simulink model "ECO_openSource"  (R2020b)
settings: Solver=FixedStepAuto  StartTime=0.0  StopTime=parECO.ref.time(end)+parECO.ref.dT  FixedStep=0.001  RelTol=1e-3  EnableMultiTasking=on
InitFcn:
  | if ~exist('parECO','var')
  |    load('parECO.mat');
  | end
  | if ~isfield(parECO,'ref')
  | 
  |    parECO.enNoise = true;
  |    parECO.enDist = true;
  |    parECO.enFB.imep = true;
  |    parECO.enFB.dpMax = true;
  |    parECO.enFB.Tevo = true;
  |    parECO.enFB.cNOx = true;
  | 
  |    parECO.ref.dT = 5;
  |    parECO.ref.imep = [  6   6   9   9   7   7 ] * 1e5
  |    parECO.ref.dpMax = [ 15   4   4   4   4   4 ] * 1e5;
  |    parECO.ref.Tevo = [  0   0   0 680   0   0 ] + 273;
  |    parECO.ref.cNOx = [100 100 100 100 100  15 ] * 1e2;
  | 
  |    parECO.ref.time  = 0 : parECO.ref.dT : parECO.ref.dT*(numel(parECO.ref.imep)-1);
  |    parECO.ref.imep  = [parECO.Reference.IMEP parECO.ref.imep(1)  parECO.ref.imep ];
  |    parECO.ref.dpMax = [parECO.Reference.dpMax parECO.ref.dpMax(1) parECO.ref.dpMax];
  |    parECO.ref.Tevo  = [parECO.Reference.Tmin parECO.ref.Tevo(1)  parECO.ref.Tevo];
  |    parECO.ref.cNOx  = [parECO.Reference.cNOx parECO.ref.cNOx(1)  parECO.ref.cNOx];
  |    parECO.ref.time  = [0 1 parECO.ref.time + parECO.ref.dT ];
  | 
  | end
undefined symbols (not defined in the file): DiscIntNeverNeededParam, parOpt, parSim
libraries: simulink x6, dspstat3 x4, dspswit3 x1, hdlsllib x1
(part 1 of 2)
settings Model: NumberOfSteps=5000  Creator=shaen  LastModifiedBy=nicolas
settings DataIOCC: ReturnWorkspaceOutputs=off
settings DebuggingCC: InheritedTsInSrcMsg=none  ArithmeticOperatorsInVariantConditions=warning
settings SFSimCC: SimUseLocalCustomCode=off  CustomCodeUndefinedFunction=UseInterfaceOnly
settings RTWCC: RTWUseLocalCustomCode=off

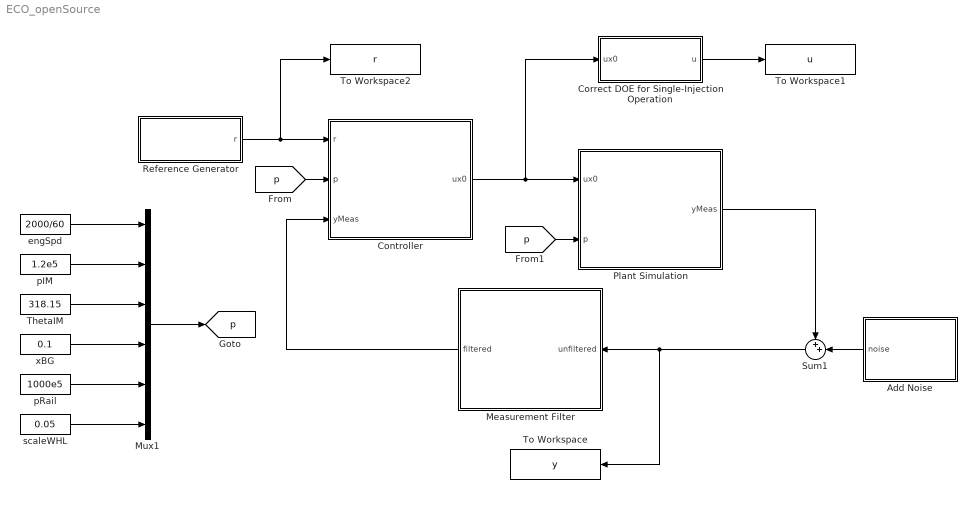
== system ECO_openSource ==
  Add Noise : Subsystem
  Controller : Subsystem  Description=test
  Correct DOE for Single-Injection Operation : Subsystem
  Measurement Filter : Subsystem
  Mux1 : Mux  Inputs=6
  Plant Simulation : Subsystem
  Reference Generator : Subsystem
  Sum1 : Sum  Inputs=++|
  ThetaIM : Constant  Value=318.15
  To Workspace : ToWorkspace  VariableName=y  SaveFormat=Timeseries  SampleTime=-1
  To Workspace1 : ToWorkspace  VariableName=u  SaveFormat=Timeseries  SampleTime=-1
  To Workspace2 : ToWorkspace  VariableName=r  SaveFormat=Timeseries  SampleTime=-1
  engSpd : Constant  Value=2000/60
  pIM : Constant  Value=1.2e5
  pRail : Constant  Value=1000e5
  scaleWHL : Constant  Value=0.05
  xBG : Constant  Value=0.1
  tag scope: p=global
  wires:
  [p] -> Plant Simulation/2(p)
  Reference Generator/1(r) -> To Workspace2/1, Controller/1(r)
  Sum1/1 -> To Workspace/1, Measurement Filter/1(unfiltered)
  pRail/1 -> Mux1/5
  Plant Simulation/1(yMeas) -> Sum1/1
  Mux1/1 -> [p]
  Correct DOE for Single-Injection Operation/1(" u ") -> To Workspace1/1
  ThetaIM/1 -> Mux1/3
  Measurement Filter/1(filtered) -> Controller/3(yMeas)
  scaleWHL/1 -> Mux1/6
  Add Noise/1(noise) -> Sum1/2
  pIM/1 -> Mux1/2
  xBG/1 -> Mux1/4
  [p] -> Controller/2(p)
  engSpd/1 -> Mux1/1
  Controller/1(ux0) -> Correct DOE for Single-Injection Operation/1(ux0), Plant Simulation/1(ux0)

== system ECO_openSource/Add Noise ==
  Gain1 : Gain  Gain=0.25*1e4
  Gain2 : Gain  Gain=2
  Gain3 : Gain  Gain=2
  Gain4 : Gain  Gain=0.15*1e5
  Mux7 : Mux
  ON/OFF : Gain  Gain=parECO.enNoise
  Random Number1 : RandomNumber  SampleTime=0.01
  Random Number2 : RandomNumber  Seed=1  SampleTime=0.01
  Random Number3 : RandomNumber  Seed=2  SampleTime=0.01
  Random Number4 : RandomNumber  Seed=1  SampleTime=0.01
  noise : Outport
  wires:
  Random Number3/1 -> Gain4/1
  Mux7/1 -> ON/OFF/1
  Random Number2/1 -> Gain3/1
  ON/OFF/1 -> noise/1
  Random Number1/1 -> Gain1/1
  Gain1/1 -> Mux7/1
  Gain4/1 -> Mux7/4
  Gain3/1 -> Mux7/3
  Random Number4/1 -> Gain2/1
  Gain2/1 -> Mux7/2

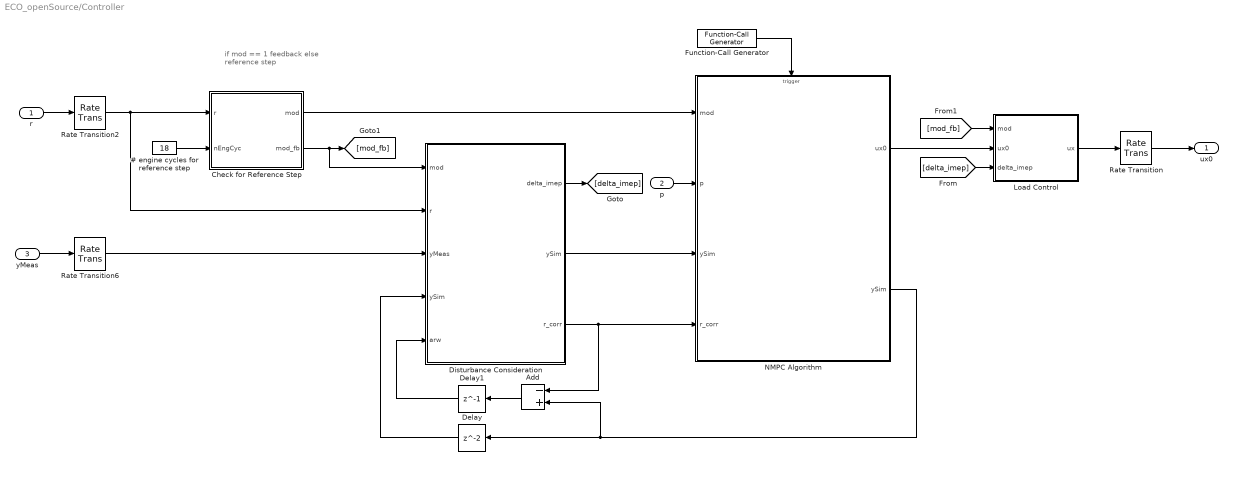
== system ECO_openSource/Controller ==
  note: if mod == 1
      | 	feedback
      | else
      | 	reference step
  r : Inport
  p : Inport  Port=2
  yMeas : Inport  Port=3
  # engine cycles for reference step : Constant  Value=18
  Add : Sum  Inputs=-+
  Check for Reference Step : Subsystem
  Delay : Delay  InitialCondition=repmat([parECO.Reference.IMEP;parECO.Reference.cNOx;parECO.Reference.Tmin;parECO.Reference.dpMax],1,2)
  Delay1 : Delay  DelayLength=1
  Disturbance Consideration : Subsystem
  Function-Call Generator : simulink/Ports & Subsystems/Function-Call Generator  sample_time=parECO.T_ECO  numberOfIterations=1  DisallowWideOutput=off
  Load Control : Subsystem
  NMPC Algorithm : Subsystem
  Rate Transition : RateTransition  InitialCondition=parECO.ux0
  Rate Transition2 : RateTransition  InitialCondition=[parECO.Reference.IMEP;parECO.Reference.cNOx;parECO.Reference.Tmin;parECO.Reference.dpMax]
  Rate Transition6 : RateTransition
  ux0 : Outport  VectorParamsAs1DForOutWhenUnconnected=off
  wires:
  Rate Transition/1 -> ux0/1
  Function-Call Generator/1 -> NMPC Algorithm/Trigger
  yMeas/1 -> Rate Transition6/1
  # engine cycles for reference step/1 -> Check for Reference Step/2(nEngCyc)
  Check for Reference Step/1(mod) -> NMPC Algorithm/1(mod)
  Rate Transition6/1 -> Disturbance Consideration/3(yMeas)
  r/1 -> Rate Transition2/1
  NMPC Algorithm/1(ux0) -> Load Control/2(ux0)
  Rate Transition2/1 -> Disturbance Consideration/2(r), Check for Reference Step/1(r)
  Add/1 -> Delay1/1
  Delay/1 -> Disturbance Consideration/4(ySim)
  Disturbance Consideration/2(" ySim ") -> NMPC Algorithm/3(" ySim ")
  Disturbance Consideration/3(r_corr) -> Add/1, NMPC Algorithm/4(r_corr)
  Load Control/1(ux) -> Rate Transition/1
  Disturbance Consideration/1(delta_imep) -> [delta_imep]
  [delta_imep] -> Load Control/3(delta_imep)
  Check for Reference Step/2(mod_fb) -> Disturbance Consideration/1(mod), [mod_fb]
  [mod_fb] -> Load Control/1(mod)
  Delay1/1 -> Disturbance Consideration/5(arw)
  p/1 -> NMPC Algorithm/2(p)
  NMPC Algorithm/2(ySim) -> Add/2, Delay/1

== system ECO_openSource/Correct DOE for Single-Injection Operation ==
  ux0 : Inport
  MATLAB Function : MATLAB Function  TreatAsAtomicUnit=on
  Selector : Selector  InputPortWidth=10  IndexOptions=Index vector (dialog)  Indices=1:4  OutputSizes=1
  " u " : Outport
  wires:
  ux0/1 -> Selector/1
  MATLAB Function/1(u) -> " u "/1
  Selector/1 -> MATLAB Function/1("u ")

== system ECO_openSource/Measurement Filter ==
  unfiltered : Inport
  Demux : Demux
  Moving Average{,1..3} (4 alike) : dspstat3/Moving Average  Method=Sliding window  SpecifyWindowLength=on  WindowLength=4  ForgettingFactor=0.9  SimulateUsing=Code generation
  Mux7 : Mux
  filtered : Outport
  wires:
  unfiltered/1 -> Demux/1
  Mux7/1 -> filtered/1
  Demux/1 -> Moving Average/1
  Moving Average/1 -> Mux7/1
  Demux/2 -> Moving Average1/1
  Moving Average1/1 -> Mux7/2
  Demux/3 -> Moving Average2/1
  Moving Average2/1 -> Mux7/3
  Demux/4 -> Moving Average3/1
  Moving Average3/1 -> Mux7/4

== system ECO_openSource/Plant Simulation ==
  ux0 : Inport
  p : Inport  Port=2
  Create Measurements : Subsystem
  Delay1 : Delay  DelayLength=1  InitialConditionSource=Input port  InitialCondition=[parOpt.u0;parSim.OP.pInt;0;0]
      settings: InputPortMap=u0,p4
  For Iterator : ForIterator  ResetStates=reset  IterationLimit=numel(parECO.ca_sim)-1  ShowIterationPort=off
  S-Function : S-Function  FunctionName=sfun_fsim  SFunctionDeploymentMode=off  EnableBusSupport=off
  dca : Constant  Value=parECO.dca_sim
  yMeas : Outport
  wires:
  S-Function/1 -> Delay1/1, Create Measurements/1(ux)  "ux"
  Delay1/1 -> S-Function/1
  Create Measurements/1(yMeas) -> yMeas/1
  S-Function/2 -> Create Measurements/2(uxdot)  "uxdot"
  S-Function/3 -> Create Measurements/3(y)  "y"
  ux0/1 -> Delay1/2
  dca/1 -> S-Function/3
  p/1 -> S-Function/2

== system ECO_openSource/Reference Generator ==
  1-D Lookup Table : Lookup_n-D  NumberOfTableDimensions=1  BreakpointsForDimension1=parECO.ref.time  Table=parECO.ref.imep  InterpMethod=Flat  ExtrapMethod=Clip  InternalRulePriority=Speed  RndMeth=Simplest  InputSameDT=on
  1-D Lookup Table1 : Lookup_n-D  NumberOfTableDimensions=1  BreakpointsForDimension1=parECO.ref.time  Table=parECO.ref.Tevo  InterpMethod=Flat  ExtrapMethod=Clip  InternalRulePriority=Speed  RndMeth=Simplest  InputSameDT=on
  1-D Lookup Table2 : Lookup_n-D  NumberOfTableDimensions=1  BreakpointsForDimension1=parECO.ref.time  Table=parECO.ref.dpMax  InterpMethod=Flat  ExtrapMethod=Clip  InternalRulePriority=Speed  RndMeth=Simplest  InputSameDT=on
  1-D Lookup Table3 : Lookup_n-D  NumberOfTableDimensions=1  BreakpointsForDimension1=parECO.ref.time  Table=parECO.ref.cNOx  InterpMethod=Flat  ExtrapMethod=Clip  InternalRulePriority=Speed  RndMeth=Simplest  InputSameDT=on
  Clock : Clock
  Mux : Mux
  r : Outport  VectorParamsAs1DForOutWhenUnconnected=off
  wires:
  1-D Lookup Table/1 -> Mux/1
  Mux/1 -> r/1
  Clock/1 -> 1-D Lookup Table1/1, 1-D Lookup Table2/1, 1-D Lookup Table3/1, 1-D Lookup Table/1
  1-D Lookup Table2/1 -> Mux/4
  1-D Lookup Table1/1 -> Mux/3
  1-D Lookup Table3/1 -> Mux/2

== system ECO_openSource/Controller/Check for Reference Step ==
  r : Inport
  nEngCyc : Inport  Port=2
  AND : Logic  AllPortsSameDT=off  OutDataTypeStr=boolean
  Add : Sum  Inputs=+-
  Constant : Constant
  Counter : dspswit3/Counter  Direction=Down  CountEvent=Rising edge  CounterSize=User defined  MaxCount=1  InitialCount=1  Output=Count  HitValue=32  ResetInput=on  SamplesPerFrame=1  Ts=-1  CntDtype=double  HitDtype=Logical
  Delay : Delay  DelayLength=4  InitialCondition=1
  Detect Change1 : simulink/Logic and Bit Operations/Detect Change  vinit=[parECO.Reference.IMEP;parECO.Reference.cNOx;parECO.Reference.Tmin;parECO.Reference.dpMax]  OutDataTypeStr=uint8
  Equal : RelationalOperator  Operator===  OutDataTypeStr=boolean  RndMeth=Simplest
  HDL Counter : hdlsllib/Sources/HDL Counter  CountType=Free running  CountInit=0  CountStep=1  CountMax=25  CountFromType=Initial value  CountFrom=0  CountResetPort=on  CountLoadPort=off  CountEnbPort=on  CountDirPort=off  CountDataType=Unsigned  CountWordLen=8  CountFracLen=0  CountSampTime=1
  NOT : Logic  Operator=NOT  AllPortsSameDT=off  OutDataTypeStr=boolean
  any : MATLAB Function  TreatAsAtomicUnit=on
  mod : Outport
  mod_fb : Outport  Port=2
  wires:
  any/1(y) -> Counter/1
  Detect Change1/1 -> any/1(u)
  Equal/1 -> HDL Counter/1, Counter/2
  Counter/1 -> Delay/1, NOT/1, AND/1, mod/1
  nEngCyc/1 -> Add/1
  r/1 -> Detect Change1/1
  NOT/1 -> HDL Counter/2
  HDL Counter/1 -> Equal/2
  Add/1 -> Equal/1
  Constant/1 -> Add/2
  Delay/1 -> AND/2
  AND/1 -> mod_fb/1

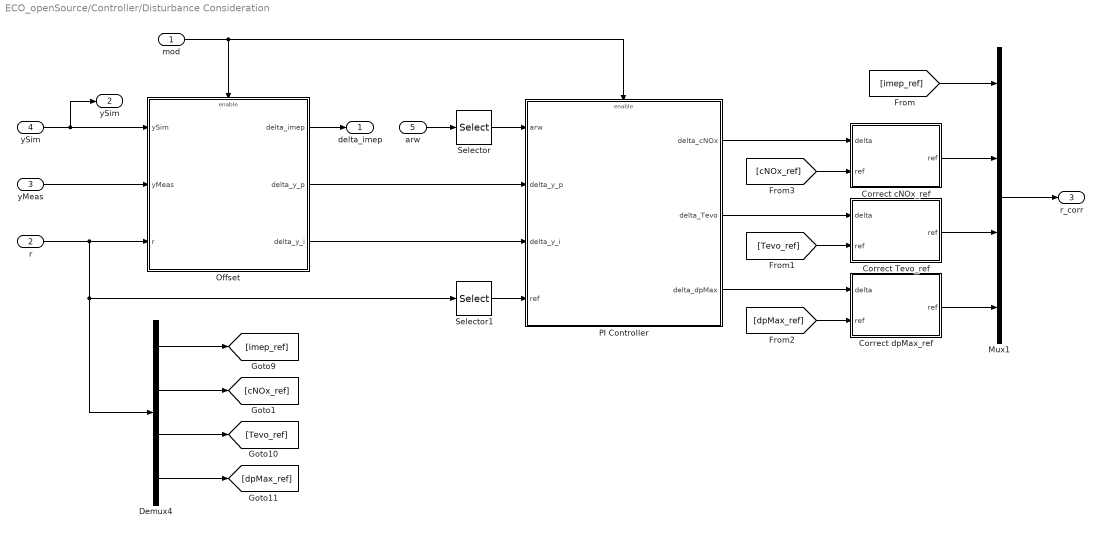
== system ECO_openSource/Controller/Disturbance Consideration ==
  mod : Inport
  r : Inport  Port=2
  yMeas : Inport  Port=3
  ySim : Inport  Port=4
  arw : Inport  Port=5
  Correct Tevo_ref : Subsystem
  Correct cNOx_ref : Subsystem
  Correct dpMax_ref : Subsystem
  Demux4 : Demux
  Mux1 : Mux
  Offset : Subsystem  TreatAsAtomicUnit=on
  PI Controller : Subsystem
  Selector : Selector  InputPortWidth=4  IndexOptions=Index vector (dialog)  Indices=2:4  OutputSizes=1
  Selector1 : Selector  InputPortWidth=4  IndexOptions=Index vector (dialog)  Indices=2:4  OutputSizes=1
  delta_imep : Outport  VectorParamsAs1DForOutWhenUnconnected=off
  " ySim " : Outport  Port=2
  r_corr : Outport  Port=3  VectorParamsAs1DForOutWhenUnconnected=off
  wires:
  yMeas/1 -> Offset/2(" yMeas ")
  Offset/2(delta_y_p) -> PI Controller/2(delta_y_p)
  Offset/3(delta_y_i) -> PI Controller/3(delta_y_i)
  ySim/1 -> Offset/1(ySim), " ySim "/1
  mod/1 -> PI Controller/Enable, Offset/Enable
  arw/1 -> Selector/1
  Mux1/1 -> r_corr/1
  [imep_ref] -> Mux1/1
  PI Controller/3(delta_dpMax) -> Correct dpMax_ref/1(delta)
  PI Controller/2(delta_Tevo) -> Correct Tevo_ref/1(delta)
  [dpMax_ref] -> Correct dpMax_ref/2(ref)
  [Tevo_ref] -> Correct Tevo_ref/2(ref)
  Demux4/1 -> [imep_ref]
  r/1 -> Selector1/1, Demux4/1, Offset/3(r)
  Demux4/4 -> [dpMax_ref]
  Demux4/3 -> [Tevo_ref]
  Demux4/2 -> [cNOx_ref]
  Correct dpMax_ref/1(" ref ") -> Mux1/4
  Correct Tevo_ref/1(" ref ") -> Mux1/3
  [cNOx_ref] -> Correct cNOx_ref/2(ref)
  PI Controller/1(delta_cNOx) -> Correct cNOx_ref/1(delta)
  Correct cNOx_ref/1(" ref ") -> Mux1/2
  Offset/1(delta_imep) -> delta_imep/1
  Selector/1 -> PI Controller/1(arw)
  Selector1/1 -> PI Controller/4(ref)

== system ECO_openSource/Controller/Load Control ==
  mod : Inport
  ux0 : Inport  Port=2
  delta_imep : Inport  Port=3
  Constant : Constant  Value=0
  Constant1 : Constant  Value=0
  Demux : Demux  Outputs=10
  Multiport Switch : MultiPortSwitch  DataPortOrder=Zero-based contiguous  Inputs=2  zeroidx=on
  Mux : Mux  Inputs=10
  PI Controller : Subsystem
  Step : Step
  Sum : Sum  Inputs=|++
  Switch : Switch  Criteria=u2 > Threshold
  activate_feedback_imep : Constant  Value=parECO.enFB.imep
  ux : Outport  VectorParamsAs1DForOutWhenUnconnected=off
  wires:
  ux0/1 -> Demux/1
  Demux/1 -> Mux/1
  Demux/2 -> Mux/2
  Demux/3 -> Mux/3
  Demux/4 -> Sum/1
  Demux/5 -> Mux/5
  Demux/6 -> Mux/6
  Demux/7 -> Mux/7
  Demux/8 -> Mux/8
  Demux/9 -> Mux/9
  Demux/10 -> Mux/10
  Sum/1 -> Mux/4
  Multiport Switch/1 -> Sum/2
  Constant/1 -> Multiport Switch/2
  Switch/1 -> Multiport Switch/1, PI Controller/1(activate_feedback_imep)
  Mux/1 -> ux/1
  delta_imep/1 -> PI Controller/2(delta_imep)
  PI Controller/1(delta_doe2) -> Multiport Switch/3
  mod/1 -> PI Controller/Enable
  activate_feedback_imep/1 -> Switch/2
  Step/1 -> Switch/1
  Constant1/1 -> Switch/3

== system ECO_openSource/Controller/NMPC Algorithm ==
  mod : Inport
  p : Inport  Port=2
  " ySim " : Inport  Port=3
  r_corr : Inport  Port=4
  Trigger : TriggerPort  TriggerType=function-call  VariantControl=Variant  SampleTimeType=periodic  SampleTime=-1  PortDimensions=1
  Delay Input for Reference Steps : Subsystem
  Delay ySim for Reference Steps : Subsystem
  Subsystem : Subsystem
  mod1 : InportShadow
  ux0 : Outport  VectorParamsAs1DForOutWhenUnconnected=off
  ySim : Outport  Port=2  VectorParamsAs1DForOutWhenUnconnected=off
  wires:
  r_corr/1 -> Subsystem/1(r_corr)
  mod/1 -> Delay Input for Reference Steps/Enable
  Subsystem/1(ux0) -> Delay Input for Reference Steps/1(ux0)
  Delay Input for Reference Steps/1(" ux0 ") -> ux0/1
  " ySim "/1 -> Subsystem/3(" ySim ")
  p/1 -> Subsystem/2(p)
  Subsystem/2(ySim) -> Delay ySim for Reference Steps/1(ySim)
  Delay ySim for Reference Steps/1(" ySim ") -> ySim/1
  mod1/1 -> Delay ySim for Reference Steps/Enable

== system ECO_openSource/Plant Simulation/Create Measurements ==
  ux : Inport
  uxdot : Inport  Port=2
  y : Inport  Port=3
  Add Disturbance : Subsystem
  Delay1 : Delay  DelayLength=1
  Max1 : MinMax  Function=max  Inputs=2
  Mux1 : Mux
  Selector1 : Selector  InputPortWidth=12  IndexOptions=Index vector (dialog)  Indices=9  OutputSizes=1
  Selector3 : Selector  InputPortWidth=10  IndexOptions=Index vector (dialog)  Indices=7  OutputSizes=1
  Selector4 : Selector  InputPortWidth=10  IndexOptions=Index vector (dialog)  Indices=5  OutputSizes=1
  Selector5 : Selector  InputPortWidth=12  IndexOptions=Index vector (dialog)  Indices=1  OutputSizes=1
  Switch : Switch  Criteria=u2 > Threshold
  en_disturbance : Constant  Value=parECO.enDist
  yMeas : Outport
  wires:
  ux/1 -> Selector3/1
  Delay1/1 -> Max1/2
  Selector3/1 -> Mux1/1
  Switch/1 -> yMeas/1
  Selector5/1 -> Mux1/3
  en_disturbance/1 -> Switch/2
  uxdot/1 -> Selector4/1
  Add Disturbance/1(disturbed) -> Switch/1
  Selector4/1 -> Max1/1
  Mux1/1 -> Add Disturbance/1(undisturbed), Switch/3
  Max1/1 -> Mux1/4, Delay1/1
  Selector1/1 -> Mux1/2
  y/1 -> Selector5/1, Selector1/1

== system ECO_openSource/Controller/Disturbance Consideration/Correct Tevo_ref ==
  delta : Inport
  ref : Inport  Port=2
  Add : Sum
  Switch : Switch  Criteria=u2 > Threshold  Threshold=parECO.Reference.Tmin
  " ref " : Outport
  wires:
  delta/1 -> Add/1
  Add/1 -> Switch/1
  Switch/1 -> " ref "/1
  ref/1 -> Add/2, Switch/3, Switch/2

== system ECO_openSource/Controller/Disturbance Consideration/Correct cNOx_ref ==
  delta : Inport
  ref : Inport  Port=2
  Add : Sum
  Switch : Switch  Threshold=parECO.Reference.cNOx
  " ref " : Outport
  wires:
  Switch/1 -> " ref "/1
  Add/1 -> Switch/3
  ref/1 -> Switch/1, Switch/2, Add/1
  delta/1 -> Add/2

== system ECO_openSource/Controller/Disturbance Consideration/Correct dpMax_ref ==
  delta : Inport
  ref : Inport  Port=2
  Add : Sum
  Switch : Switch  Threshold=parECO.Reference.dpMax
  " ref " : Outport
  wires:
  delta/1 -> Add/2
  ref/1 -> Add/1, Switch/1, Switch/2
  Add/1 -> Switch/3
  Switch/1 -> " ref "/1

== system ECO_openSource/Controller/Disturbance Consideration/Offset ==
  ySim : Inport
  " yMeas " : Inport  Port=2
  r : Inport  Port=3
  Enable : EnablePort
  Integrational Offset : Subsystem
  Proportional Offset : Subsystem
  yMeas : InportShadow  Port=2
  delta_imep : Outport  VectorParamsAs1DForOutWhenUnconnected=off
  delta_y_p : Outport  Port=2
  delta_y_i : Outport  Port=3
  wires:
  ySim/1 -> Proportional Offset/1(ySim)
  " yMeas "/1 -> Integrational Offset/2(yMeas)
  r/1 -> Integrational Offset/1(r)
  yMeas/1 -> Proportional Offset/2(yMeas)
  Integrational Offset/1(delta_y_i) -> delta_y_i/1
  Proportional Offset/1(delta_y_p) -> delta_y_p/1
  Integrational Offset/2(delta_imep) -> delta_imep/1

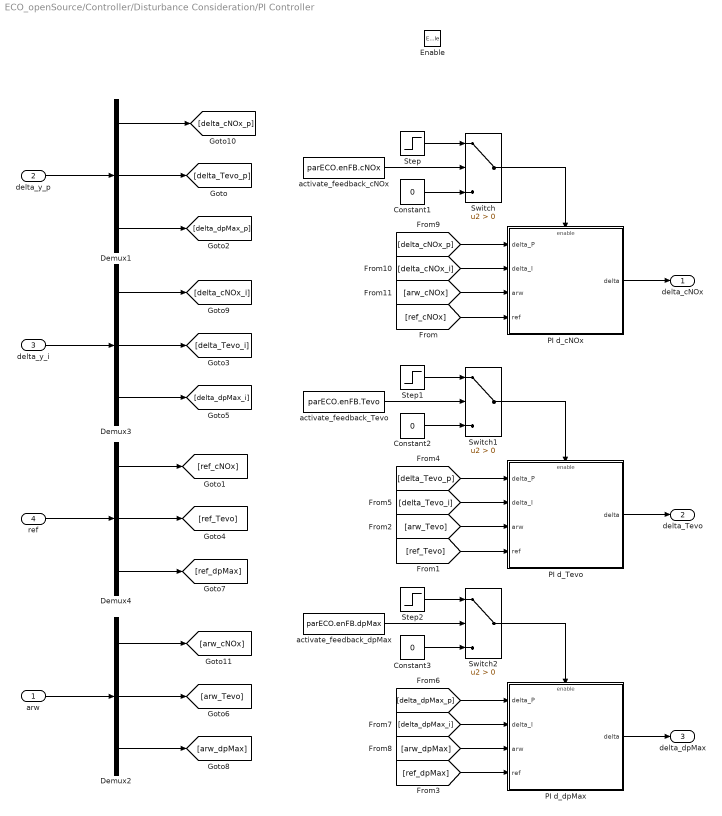
== system ECO_openSource/Controller/Disturbance Consideration/PI Controller ==
  arw : Inport
  delta_y_p : Inport  Port=2
  delta_y_i : Inport  Port=3
  ref : Inport  Port=4
  Enable : EnablePort
  Constant1 : Constant  Value=0
  Constant2 : Constant  Value=0
  Constant3 : Constant  Value=0
  Demux{1..4} (4 alike) : Demux  Outputs=3
  PI d_Tevo : Subsystem
  PI d_cNOx : Subsystem
  PI d_dpMax : Subsystem
  Step : Step
  Step1 : Step
  Step2 : Step
  Switch : Switch  Criteria=u2 > Threshold
  Switch1 : Switch  Criteria=u2 > Threshold
  Switch2 : Switch  Criteria=u2 > Threshold
  activate_feedback_Tevo : Constant  Value=parECO.enFB.Tevo
  activate_feedback_cNOx : Constant  Value=parECO.enFB.cNOx
  activate_feedback_dpMax : Constant  Value=parECO.enFB.dpMax
  delta_cNOx : Outport
  delta_Tevo : Outport  Port=2
  delta_dpMax : Outport  Port=3
  wires:
  delta_y_p/1 -> Demux1/1
  delta_y_i/1 -> Demux3/1
  [delta_Tevo_i] -> PI d_Tevo/2(delta_I)
  [delta_Tevo_p] -> PI d_Tevo/1(delta_P)
  [delta_dpMax_i] -> PI d_dpMax/2(delta_I)
  [delta_dpMax_p] -> PI d_dpMax/1(delta_P)
  PI d_Tevo/1(delta) -> delta_Tevo/1
  PI d_dpMax/1(delta) -> delta_dpMax/1
  [arw_Tevo] -> PI d_Tevo/3(arw)
  arw/1 -> Demux2/1
  [arw_dpMax] -> PI d_dpMax/3(arw)
  Switch2/1 -> PI d_dpMax/Enable
  [arw_cNOx] -> PI d_cNOx/3(arw)
  [delta_cNOx_i] -> PI d_cNOx/2(delta_I)
  Switch/1 -> PI d_cNOx/Enable
  PI d_cNOx/1(delta) -> delta_cNOx/1
  [delta_cNOx_p] -> PI d_cNOx/1(delta_P)
  Step/1 -> Switch/1
  activate_feedback_cNOx/1 -> Switch/2
  Constant1/1 -> Switch/3
  Step1/1 -> Switch1/1
  Constant2/1 -> Switch1/3
  activate_feedback_Tevo/1 -> Switch1/2
  Step2/1 -> Switch2/1
  Constant3/1 -> Switch2/3
  activate_feedback_dpMax/1 -> Switch2/2
  Switch1/1 -> PI d_Tevo/Enable
  ref/1 -> Demux4/1
  [ref_cNOx] -> PI d_cNOx/4(ref)
  [ref_Tevo] -> PI d_Tevo/4(ref)
  [ref_dpMax] -> PI d_dpMax/4(ref)
  Demux1/3 -> [delta_dpMax_p]
  Demux1/2 -> [delta_Tevo_p]
  Demux1/1 -> [delta_cNOx_p]
  Demux3/3 -> [delta_dpMax_i]
  Demux3/2 -> [delta_Tevo_i]
  Demux3/1 -> [delta_cNOx_i]
  Demux2/3 -> [arw_dpMax]
  Demux2/2 -> [arw_Tevo]
  Demux2/1 -> [arw_cNOx]
  Demux4/3 -> [ref_dpMax]
  Demux4/2 -> [ref_Tevo]
  Demux4/1 -> [ref_cNOx]

== system ECO_openSource/Controller/Load Control/PI Controller ==
  activate_feedback_imep : Inport
  delta_imep : Inport  Port=2
  Enable : EnablePort
  Ki : Constant  Value=1.1e-4  VectorParams1D=off
  Kp : Constant  Value=1.5e-4  VectorParams1D=off
  PI Controller imep : Subsystem
  delta_doe2 : Outport  VectorParamsAs1DForOutWhenUnconnected=off
  wires:
  Ki/1 -> PI Controller imep/3(I)
  delta_imep/1 -> PI Controller imep/1(delta_P)
  Kp/1 -> PI Controller imep/2(P)
  PI Controller imep/1(delta) -> delta_doe2/1
  activate_feedback_imep/1 -> PI Controller imep/Enable

== system ECO_openSource/Controller/NMPC Algorithm/Delay Input for Reference Steps ==
  ux0 : Inport
  Enable : EnablePort
  " ux0 " : Outport
  wires:
  ux0/1 -> " ux0 "/1

== system ECO_openSource/Controller/NMPC Algorithm/Delay ySim for Reference Steps ==
  ySim : Inport
  Enable : EnablePort
  " ySim " : Outport
  wires:
  ySim/1 -> " ySim "/1

== system ECO_openSource/Controller/NMPC Algorithm/Subsystem ==
  r_corr : Inport
  p : Inport  Port=2
  " ySim " : Inport  Port=3
  Algorithm : Subsystem
  For Iterator : ForIterator  IterationLimit=parECO.nIter  ShowIterationPort=off
  Limit Reference and Reference Changes : Subsystem
  ux0 : Outport  VectorParamsAs1DForOutWhenUnconnected=off
  ySim : Outport  Port=2  VectorParamsAs1DForOutWhenUnconnected=off
  wires:
  Algorithm/1(ux0) -> ux0/1
  r_corr/1 -> Limit Reference and Reference Changes/1(r_corr)
  Limit Reference and Reference Changes/1(r_corr_limited) -> Algorithm/2(r_corr)
  " ySim "/1 -> Limit Reference and Reference Changes/2(" ySim ")
  p/1 -> Algorithm/1(p)
  Algorithm/2(ySim) -> ySim/1

== system ECO_openSource/Plant Simulation/Create Measurements/Add Disturbance ==
  undisturbed : Inport
  Add : Sum
  Add2 : Sum
  Add3 : Sum
  Demux : Demux
  Mux : Mux
  Product : Product
  Tevo_offset : Constant  Value=10
  cNOx_offset : Constant  Value=30
  dpMax_offset : Constant  Value=0.3e5
  imep_offset : Constant  Value=1.1
  disturbed : Outport
  wires:
  imep_offset/1 -> Product/2
  Tevo_offset/1 -> Add/2
  Demux/1 -> Product/1
  dpMax_offset/1 -> Add2/2
  undisturbed/1 -> Demux/1
  Product/1 -> Mux/1
  Mux/1 -> disturbed/1
  Demux/4 -> Add2/1
  Add2/1 -> Mux/4
  Add/1 -> Mux/3
  Demux/3 -> Add/1
  Demux/2 -> Add3/1
  Add3/1 -> Mux/2
  cNOx_offset/1 -> Add3/2

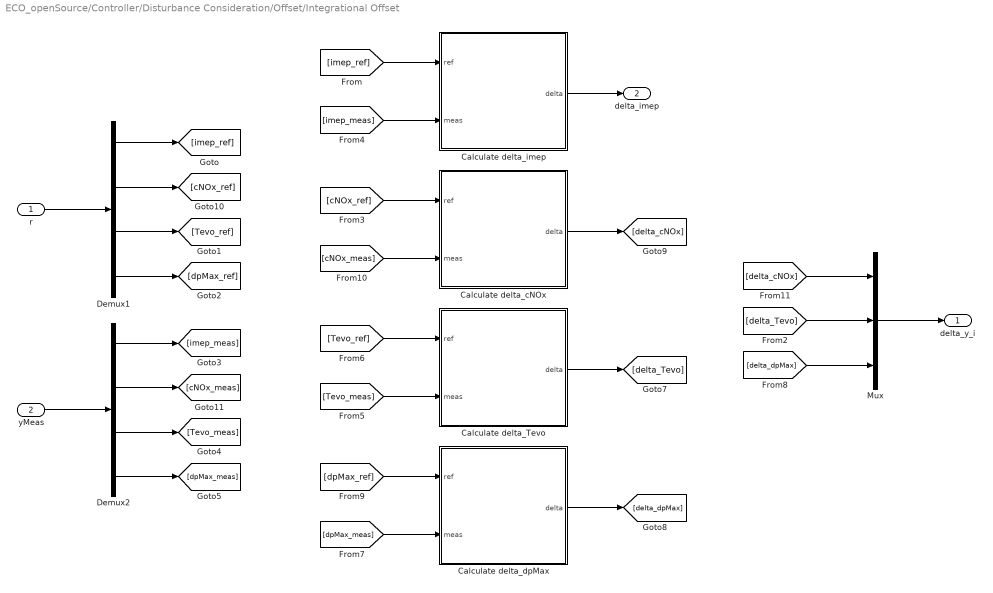
== system ECO_openSource/Controller/Disturbance Consideration/Offset/Integrational Offset ==
  r : Inport
  yMeas : Inport  Port=2
  Calculate delta_Tevo : Subsystem  TreatAsAtomicUnit=on
  Calculate delta_cNOx : Subsystem  TreatAsAtomicUnit=on
  Calculate delta_dpMax : Subsystem  TreatAsAtomicUnit=on
  Calculate delta_imep : Subsystem  TreatAsAtomicUnit=on
  Demux1 : Demux
  Demux2 : Demux
  Mux : Mux  Inputs=3
  delta_y_i : Outport  Tag=p_im  VectorParamsAs1DForOutWhenUnconnected=off
  delta_imep : Outport  Port=2  VectorParamsAs1DForOutWhenUnconnected=off
  wires:
  Demux1/1 -> [imep_ref]
  r/1 -> Demux1/1
  Mux/1 -> delta_y_i/1
  [imep_ref] -> Calculate delta_imep/1(ref)
  [imep_meas] -> Calculate delta_imep/2(meas)
  [Tevo_meas] -> Calculate delta_Tevo/2(meas)
  [Tevo_ref] -> Calculate delta_Tevo/1(ref)
  [dpMax_meas] -> Calculate delta_dpMax/2(meas)
  [dpMax_ref] -> Calculate delta_dpMax/1(ref)
  Calculate delta_imep/1(delta) -> delta_imep/1
  Calculate delta_Tevo/1(delta) -> [delta_Tevo]
  Calculate delta_dpMax/1(delta) -> [delta_dpMax]
  yMeas/1 -> Demux2/1
  Demux2/1 -> [imep_meas]
  [cNOx_ref] -> Calculate delta_cNOx/1(ref)
  [cNOx_meas] -> Calculate delta_cNOx/2(meas)
  Calculate delta_cNOx/1(delta) -> [delta_cNOx]
  Demux1/3 -> [Tevo_ref]
  Demux1/4 -> [dpMax_ref]
  Demux1/2 -> [cNOx_ref]
  Demux2/2 -> [cNOx_meas]
  Demux2/3 -> [Tevo_meas]
  Demux2/4 -> [dpMax_meas]
  [delta_dpMax] -> Mux/3
  [delta_Tevo] -> Mux/2
  [delta_cNOx] -> Mux/1

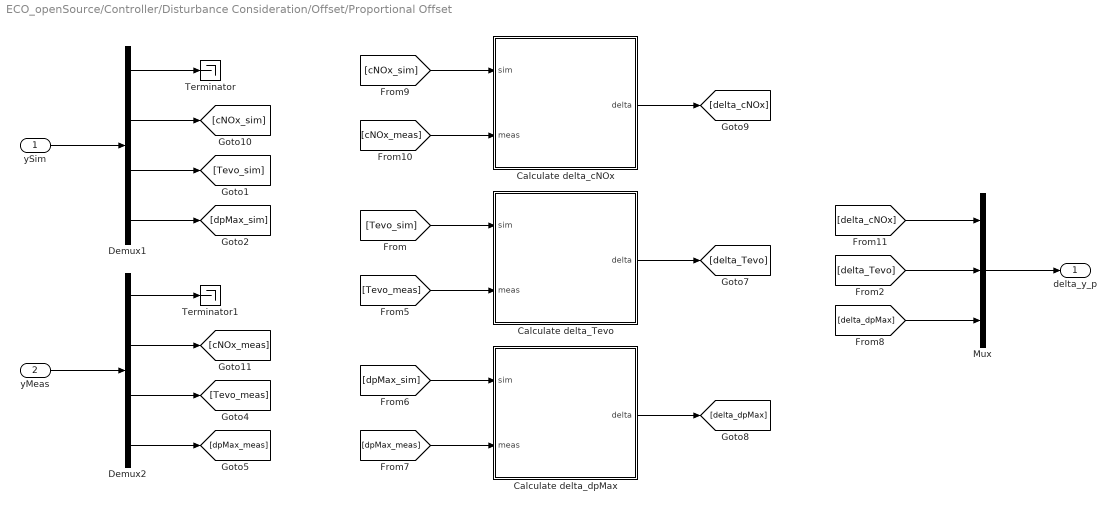
== system ECO_openSource/Controller/Disturbance Consideration/Offset/Proportional Offset ==
  ySim : Inport
  yMeas : Inport  Port=2
  Calculate delta_Tevo : Subsystem  TreatAsAtomicUnit=on
  Calculate delta_cNOx : Subsystem  TreatAsAtomicUnit=on
  Calculate delta_dpMax : Subsystem  TreatAsAtomicUnit=on
  Demux1 : Demux
  Demux2 : Demux
  Mux : Mux  Inputs=3
  Terminator : Terminator
  Terminator1 : Terminator
  delta_y_p : Outport  Tag=p_im  VectorParamsAs1DForOutWhenUnconnected=off
  wires:
  Demux1/1 -> Terminator/1
  ySim/1 -> Demux1/1
  Mux/1 -> delta_y_p/1
  [Tevo_meas] -> Calculate delta_Tevo/2(meas)
  [Tevo_sim] -> Calculate delta_Tevo/1(sim)
  [dpMax_meas] -> Calculate delta_dpMax/2(meas)
  [dpMax_sim] -> Calculate delta_dpMax/1(sim)
  Calculate delta_Tevo/1(delta) -> [delta_Tevo]
  Calculate delta_dpMax/1(delta) -> [delta_dpMax]
  yMeas/1 -> Demux2/1
  Demux2/1 -> Terminator1/1
  [cNOx_sim] -> Calculate delta_cNOx/1(sim)
  [cNOx_meas] -> Calculate delta_cNOx/2(meas)
  Calculate delta_cNOx/1(delta) -> [delta_cNOx]
  Demux1/3 -> [Tevo_sim]
  Demux1/4 -> [dpMax_sim]
  Demux1/2 -> [cNOx_sim]
  Demux2/2 -> [cNOx_meas]
  Demux2/3 -> [Tevo_meas]
  Demux2/4 -> [dpMax_meas]
  [delta_dpMax] -> Mux/3
  [delta_Tevo] -> Mux/2
  [delta_cNOx] -> Mux/1

== system ECO_openSource/Controller/Disturbance Consideration/PI Controller/PI d_Tevo ==
  delta_P : Inport
  delta_I : Inport  Port=2
  arw : Inport  Port=3
  ref : Inport  Port=4
  Enable : EnablePort
  Ki : Constant  Value=0.7  VectorParams1D=off
  Kp : Constant  Value=0.7  VectorParams1D=off
  PI Controller Tevo : Subsystem
  delta : Outport
  wires:
  delta_I/1 -> PI Controller Tevo/2(delta_I)
  Kp/1 -> PI Controller Tevo/3(P)
  arw/1 -> PI Controller Tevo/5(arw)
  Ki/1 -> PI Controller Tevo/4(I)
  PI Controller Tevo/1(delta) -> delta/1
  delta_P/1 -> PI Controller Tevo/1(delta_P)
  ref/1 -> PI Controller Tevo/6(ref)

== system ECO_openSource/Controller/Disturbance Consideration/PI Controller/PI d_cNOx ==
  delta_P : Inport
  delta_I : Inport  Port=2
  arw : Inport  Port=3
  ref : Inport  Port=4
  Enable : EnablePort
  Ki : Constant  Value=0.7  VectorParams1D=off
  Kp : Constant  Value=0.7  VectorParams1D=off
  PI Controller Tevo : Subsystem
  delta : Outport
  wires:
  delta_I/1 -> PI Controller Tevo/2(delta_I)
  Kp/1 -> PI Controller Tevo/3(P)
  arw/1 -> PI Controller Tevo/5(arw)
  Ki/1 -> PI Controller Tevo/4(I)
  PI Controller Tevo/1(delta) -> delta/1
  delta_P/1 -> PI Controller Tevo/1(delta_P)
  ref/1 -> PI Controller Tevo/6(ref)

== system ECO_openSource/Controller/Disturbance Consideration/PI Controller/PI d_dpMax ==
  delta_P : Inport
  delta_I : Inport  Port=2
  arw : Inport  Port=3
  ref : Inport  Port=4
  Enable : EnablePort
  Ki : Constant  Value=0.7  VectorParams1D=off
  Kp : Constant  Value=0.7  VectorParams1D=off
  PI Controller Tevo : Subsystem
  delta : Outport
  wires:
  delta_I/1 -> PI Controller Tevo/2(delta_I)
  Kp/1 -> PI Controller Tevo/3(P)
  arw/1 -> PI Controller Tevo/5(arw)
  Ki/1 -> PI Controller Tevo/4(I)
  PI Controller Tevo/1(delta) -> delta/1
  delta_P/1 -> PI Controller Tevo/1(delta_P)
  ref/1 -> PI Controller Tevo/6(ref)

== system ECO_openSource/Controller/Load Control/PI Controller/PI Controller imep ==
  delta_P : Inport
  P : Inport  Port=2
  I : Inport  Port=3
  Enable : EnablePort
  " " : DiscreteIntegrator  DisableCoverage=on  IntegratorMethod=Accumulation: Forward Euler  SampleTime=-1  ICPrevOutput=DiscIntNeverNeededParam  ICPrevScaledInput=DiscIntNeverNeededParam
  Product1 : Product
  Product2 : Product
  Sum3 : Sum  Inputs=++|
  delta : Outport  InitialOutput=0  VectorParamsAs1DForOutWhenUnconnected=off
  wires:
  I/1 -> Product1/2
  Sum3/1 -> delta/1
  P/1 -> Product2/2
  " "/1 -> Sum3/2
  delta_P/1 -> Product1/1, Product2/1
  Product2/1 -> Sum3/1
  Product1/1 -> " "/1

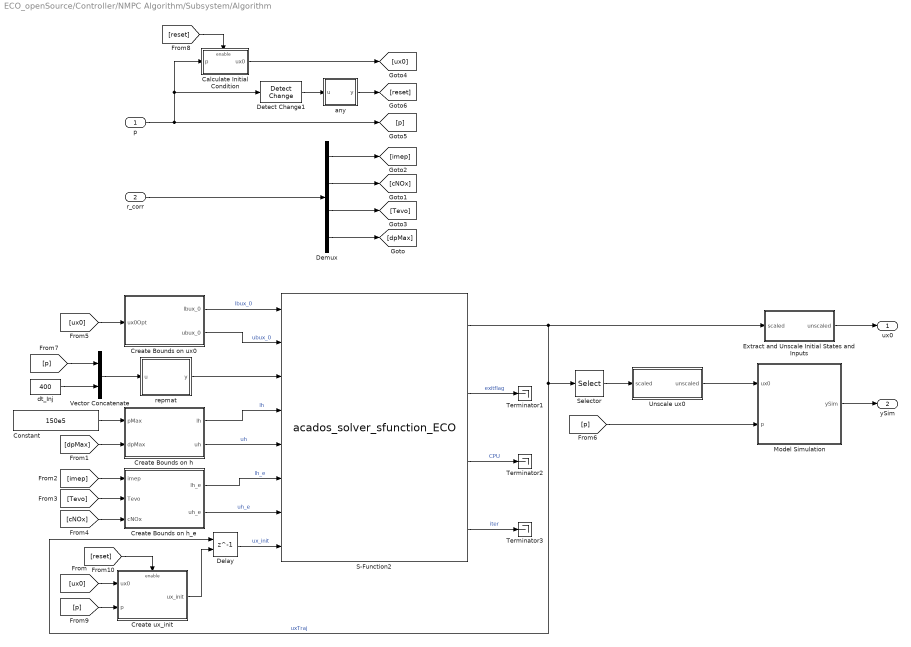
== system ECO_openSource/Controller/NMPC Algorithm/Subsystem/Algorithm ==
  p : Inport
  r_corr : Inport  Port=2
  Calculate Initial Condition : Subsystem  TreatAsAtomicUnit=on
  Constant : Constant  Value=150e5
  Create Bounds on h : Subsystem
  Create Bounds on h_e : Subsystem
  Create Bounds on ux0 : Subsystem
  Create ux_init : Subsystem
  Delay : Delay  DelayLength=1  InitialConditionSource=Input port  InitialCondition=parECO.x_init
      settings: InputPortMap=u0,p4
  Demux : Demux
  Detect Change1 : simulink/Logic and Bit Operations/Detect Change  vinit=0  OutDataTypeStr=boolean
  Extract and Unscale Initial States and Inputs : Subsystem
  Model Simulation : Subsystem
  S-Function2 : S-Function  FunctionName=acados_solver_sfunction_ECO  SFunctionDeploymentMode=off  EnableBusSupport=off
  Selector : Selector  IndexOptions=Index vector (dialog)  Indices=1:10  OutputSizes=1
  Terminator1 : Terminator
  Terminator2 : Terminator
  Terminator3 : Terminator
  Unscale ux0 : Subsystem
  Vector Concatenate : Concatenate
  any : MATLAB Function  TreatAsAtomicUnit=on
  dt_Inj : Constant  Value=400
  repmat : MATLAB Function  TreatAsAtomicUnit=on  mask{N=parECO.N+1}
  ux0 : Outport
  ySim : Outport  Port=2  VectorParamsAs1DForOutWhenUnconnected=off
  wires:
  Extract and Unscale Initial States and Inputs/1(unscaled) -> ux0/1
  Demux/1 -> [imep]
  r_corr/1 -> Demux/1
  Constant/1 -> Create Bounds on h/1(pMax)
  [dpMax] -> Create Bounds on h/2(dpMax)
  [imep] -> Create Bounds on h_e/1(imep)
  [Tevo] -> Create Bounds on h_e/2(Tevo)
  [ux0] -> Create Bounds on ux0/1(ux0Opt)
  Create ux_init/1(ux_init) -> Delay/2
  [ux0] -> Create ux_init/1(ux0)
  S-Function2/1 -> Delay/1, Selector/1, Extract and Unscale Initial States and Inputs/1(scaled)  "uxTraj"
  Create Bounds on ux0/1(lbux_0) -> S-Function2/1  "lbux_0"
  Create Bounds on ux0/2(ubux_0) -> S-Function2/2  "ubux_0"
  S-Function2/2 -> Terminator1/1  "exitflag"
  S-Function2/3 -> Terminator2/1  "CPU"
  S-Function2/4 -> Terminator3/1  "iter"
  Calculate Initial Condition/1(ux0) -> [ux0]
  Demux/4 -> [dpMax]
  Demux/3 -> [Tevo]
  Demux/2 -> [cNOx]
  [cNOx] -> Create Bounds on h_e/3(cNOx)
  Delay/1 -> S-Function2/8  "ux_init"
  Create Bounds on h_e/2(uh_e) -> S-Function2/7  "uh_e"
  Create Bounds on h_e/1(lh_e) -> S-Function2/6  "lh_e"
  Create Bounds on h/2(uh) -> S-Function2/5  "uh"
  Create Bounds on h/1(lh) -> S-Function2/4  "lh"
  [p] -> Vector Concatenate/1
  Vector Concatenate/1 -> repmat/1(u)
  dt_Inj/1 -> Vector Concatenate/2
  repmat/1(y) -> S-Function2/3
  Selector/1 -> Unscale ux0/1(scaled)
  [p] -> Model Simulation/2(p)
  any/1(y) -> [reset]
  Detect Change1/1 -> any/1(u)
  p/1 -> [p], Calculate Initial Condition/1(p), Detect Change1/1
  [reset] -> Calculate Initial Condition/Enable
  [p] -> Create ux_init/2(p)
  [reset] -> Create ux_init/Enable
  Model Simulation/1(ySim) -> ySim/1
  Unscale ux0/1(unscaled) -> Model Simulation/1(ux0)

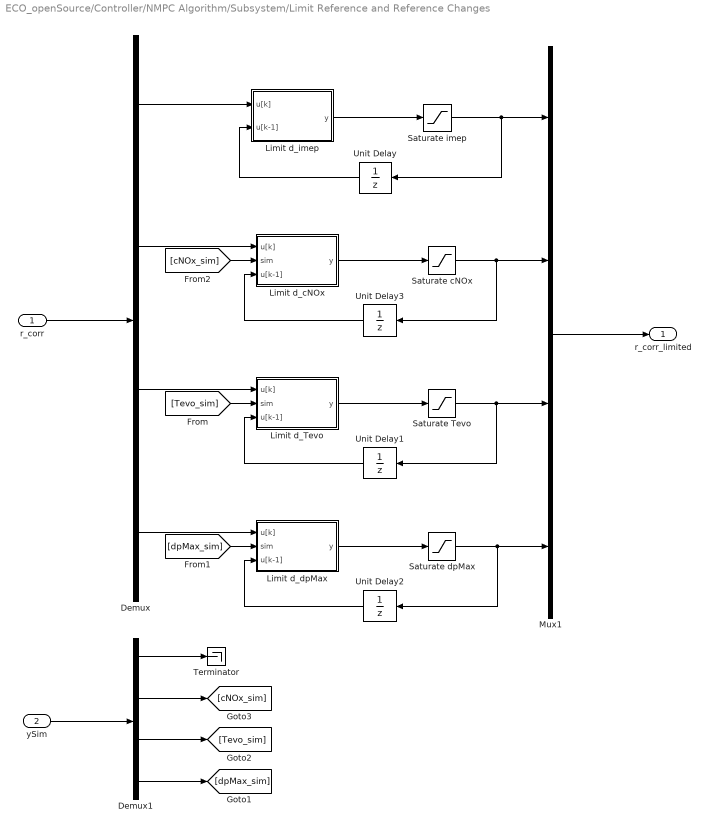
== system ECO_openSource/Controller/NMPC Algorithm/Subsystem/Limit Reference and Reference Changes ==
  r_corr : Inport
  " ySim " : Inport  Port=2
  Demux : Demux
  Demux1 : Demux
  Limit d_Tevo : Subsystem
  Limit d_cNOx : Subsystem
  Limit d_dpMax : Subsystem
  Limit d_imep : Subsystem
  Mux1 : Mux
  Saturate Tevo : Saturate  UpperLimit=1e4  LowerLimit=273
  Saturate cNOx : Saturate  UpperLimit=1e4  LowerLimit=0
  Saturate dpMax : Saturate  UpperLimit=15e5  LowerLimit=3e5
  Saturate imep : Saturate  UpperLimit=10e5  LowerLimit=2e5
  Terminator : Terminator
  Unit Delay : UnitDelay  InitialCondition=parECO.Reference.IMEP  SampleTime=-1  HasFrameUpgradeWarning=on
  Unit Delay1 : UnitDelay  InitialCondition=parECO.Reference.Tmin  SampleTime=-1  HasFrameUpgradeWarning=on
  Unit Delay2 : UnitDelay  InitialCondition=parECO.Reference.dpMax  SampleTime=-1  HasFrameUpgradeWarning=on
  Unit Delay3 : UnitDelay  InitialCondition=parECO.Reference.cNOx  SampleTime=-1  HasFrameUpgradeWarning=on
  r_corr_limited : Outport
  wires:
  r_corr/1 -> Demux/1
  Mux1/1 -> r_corr_limited/1
  Saturate imep/1 -> Unit Delay/1, Mux1/1
  Saturate Tevo/1 -> Mux1/3, Unit Delay1/1
  Saturate dpMax/1 -> Unit Delay2/1, Mux1/4
  Unit Delay/1 -> Limit d_imep/2(u[k-1])
  Limit d_imep/1(y) -> Saturate imep/1
  Demux/1 -> Limit d_imep/1(u[k])
  Limit d_Tevo/1(y) -> Saturate Tevo/1
  Unit Delay1/1 -> Limit d_Tevo/3(u[k-1])
  Limit d_dpMax/1(y) -> Saturate dpMax/1
  Unit Delay2/1 -> Limit d_dpMax/3(u[k-1])
  [Tevo_sim] -> Limit d_Tevo/2(sim)
  " ySim "/1 -> Demux1/1
  [dpMax_sim] -> Limit d_dpMax/2(sim)
  Demux1/1 -> Terminator/1
  Demux1/4 -> [dpMax_sim]
  Demux1/3 -> [Tevo_sim]
  Demux1/2 -> [cNOx_sim]
  Demux/3 -> Limit d_Tevo/1(u[k])
  Demux/4 -> Limit d_dpMax/1(u[k])
  Demux/2 -> Limit d_cNOx/1(u[k])
  Unit Delay3/1 -> Limit d_cNOx/3(u[k-1])
  Saturate cNOx/1 -> Mux1/2, Unit Delay3/1
  Limit d_cNOx/1(y) -> Saturate cNOx/1
  [cNOx_sim] -> Limit d_cNOx/2(sim)

== system ECO_openSource/Controller/Disturbance Consideration/Offset/Integrational Offset/Calculate delta_Tevo ==
  ref : Inport
  meas : Inport  Port=2
  Add : Sum  Inputs=-+
  delta : Outport
  wires:
  meas/1 -> Add/1
  ref/1 -> Add/2
  Add/1 -> delta/1

== system ECO_openSource/Controller/Disturbance Consideration/Offset/Integrational Offset/Calculate delta_cNOx ==
  ref : Inport
  meas : Inport  Port=2
  Add : Sum  Inputs=+-
  delta : Outport
  wires:
  ref/1 -> Add/1
  meas/1 -> Add/2
  Add/1 -> delta/1

== system ECO_openSource/Controller/Disturbance Consideration/Offset/Integrational Offset/Calculate delta_dpMax ==
  ref : Inport
  meas : Inport  Port=2
  Add : Sum  Inputs=+-
  delta : Outport
  wires:
  ref/1 -> Add/1
  meas/1 -> Add/2
  Add/1 -> delta/1

== system ECO_openSource/Controller/Disturbance Consideration/Offset/Integrational Offset/Calculate delta_imep ==
  ref : Inport
  meas : Inport  Port=2
  Add : Sum  Inputs=+-
  delta : Outport
  wires:
  ref/1 -> Add/1
  meas/1 -> Add/2
  Add/1 -> delta/1

== system ECO_openSource/Controller/Disturbance Consideration/Offset/Proportional Offset/Calculate delta_Tevo ==
  sim : Inport
  meas : Inport  Port=2
  Add : Sum  Inputs=+-
  delta : Outport
  wires:
  sim/1 -> Add/1
  meas/1 -> Add/2
  Add/1 -> delta/1

== system ECO_openSource/Controller/Disturbance Consideration/Offset/Proportional Offset/Calculate delta_cNOx ==
  sim : Inport
  meas : Inport  Port=2
  Add : Sum  Inputs=+-
  delta : Outport
  wires:
  sim/1 -> Add/1
  meas/1 -> Add/2
  Add/1 -> delta/1

== system ECO_openSource/Controller/Disturbance Consideration/Offset/Proportional Offset/Calculate delta_dpMax ==
  sim : Inport
  meas : Inport  Port=2
  Add : Sum  Inputs=+-
  delta : Outport
  wires:
  sim/1 -> Add/1
  meas/1 -> Add/2
  Add/1 -> delta/1

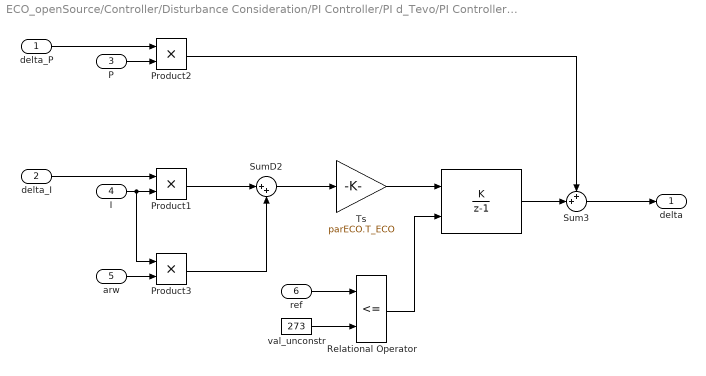
== system ECO_openSource/Controller/Disturbance Consideration/PI Controller/PI d_Tevo/PI Controller Tevo ==
  delta_P : Inport
  delta_I : Inport  Port=2
  P : Inport  Port=3
  I : Inport  Port=4
  arw : Inport  Port=5
  ref : Inport  Port=6
  " " : DiscreteIntegrator  DisableCoverage=on  IntegratorMethod=Accumulation: Forward Euler  ExternalReset=level  SampleTime=-1  ICPrevOutput=DiscIntNeverNeededParam  ICPrevScaledInput=DiscIntNeverNeededParam
  Product1 : Product
  Product2 : Product
  Product3 : Product
  Relational Operator : RelationalOperator  Operator=<=  OutDataTypeStr=boolean  RndMeth=Simplest
  Sum3 : Sum  Inputs=++|
  SumD2 : Sum  DisableCoverage=on  Inputs=|++
  Ts : Gain  Gain=parECO.T_ECO
  val_unconstr : Constant  Value=273
  delta : Outport  InitialOutput=0  VectorParamsAs1DForOutWhenUnconnected=off
  wires:
  I/1 -> Product3/1, Product1/2
  Sum3/1 -> delta/1
  P/1 -> Product2/2
  " "/1 -> Sum3/2
  delta_I/1 -> Product1/1
  Product2/1 -> Sum3/1
  SumD2/1 -> Ts/1
  arw/1 -> Product3/2
  Product3/1 -> SumD2/2
  delta_P/1 -> Product2/1
  Product1/1 -> SumD2/1
  Ts/1 -> " "/1
  ref/1 -> Relational Operator/1
  val_unconstr/1 -> Relational Operator/2
  Relational Operator/1 -> " "/2

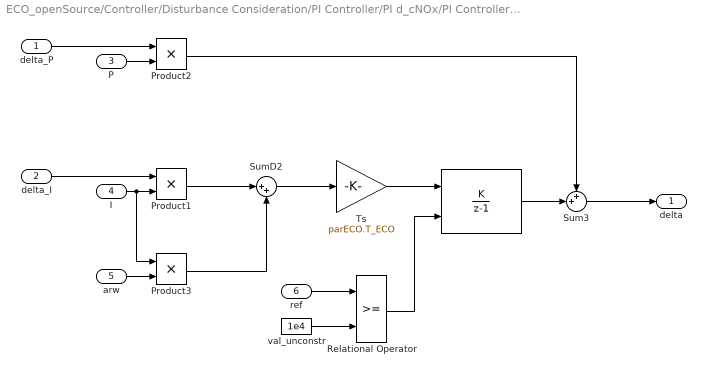
== system ECO_openSource/Controller/Disturbance Consideration/PI Controller/PI d_cNOx/PI Controller Tevo ==
  delta_P : Inport
  delta_I : Inport  Port=2
  P : Inport  Port=3
  I : Inport  Port=4
  arw : Inport  Port=5
  ref : Inport  Port=6
  " " : DiscreteIntegrator  DisableCoverage=on  IntegratorMethod=Accumulation: Forward Euler  ExternalReset=level  SampleTime=-1  ICPrevOutput=DiscIntNeverNeededParam  ICPrevScaledInput=DiscIntNeverNeededParam
  Product1 : Product
  Product2 : Product
  Product3 : Product
  Relational Operator : RelationalOperator  OutDataTypeStr=boolean  RndMeth=Simplest
  Sum3 : Sum  Inputs=++|
  SumD2 : Sum  DisableCoverage=on  Inputs=|++
  Ts : Gain  Gain=parECO.T_ECO
  val_unconstr : Constant  Value=1e4
  delta : Outport  InitialOutput=0  VectorParamsAs1DForOutWhenUnconnected=off
  wires:
  I/1 -> Product3/1, Product1/2
  Sum3/1 -> delta/1
  P/1 -> Product2/2
  " "/1 -> Sum3/2
  delta_I/1 -> Product1/1
  Product2/1 -> Sum3/1
  SumD2/1 -> Ts/1
  arw/1 -> Product3/2
  Product3/1 -> SumD2/2
  delta_P/1 -> Product2/1
  Product1/1 -> SumD2/1
  Ts/1 -> " "/1
  ref/1 -> Relational Operator/1
  val_unconstr/1 -> Relational Operator/2
  Relational Operator/1 -> " "/2

== system ECO_openSource/Controller/Disturbance Consideration/PI Controller/PI d_dpMax/PI Controller Tevo ==
  delta_P : Inport
  delta_I : Inport  Port=2
  P : Inport  Port=3
  I : Inport  Port=4
  arw : Inport  Port=5
  ref : Inport  Port=6
  " " : DiscreteIntegrator  DisableCoverage=on  IntegratorMethod=Accumulation: Forward Euler  ExternalReset=level  SampleTime=-1  ICPrevOutput=DiscIntNeverNeededParam  ICPrevScaledInput=DiscIntNeverNeededParam
  Product1 : Product
  Product2 : Product
  Product3 : Product
  Relational Operator : RelationalOperator  OutDataTypeStr=boolean  RndMeth=Simplest
  Sum3 : Sum  Inputs=++|
  SumD2 : Sum  DisableCoverage=on  Inputs=|++
  Ts : Gain  Gain=parECO.T_ECO
  val_unconstr : Constant  Value=15e5
  delta : Outport  InitialOutput=0  VectorParamsAs1DForOutWhenUnconnected=off
  wires:
  I/1 -> Product3/1, Product1/2
  Sum3/1 -> delta/1
  P/1 -> Product2/2
  " "/1 -> Sum3/2
  delta_I/1 -> Product1/1
  Product2/1 -> Sum3/1
  SumD2/1 -> Ts/1
  arw/1 -> Product3/2
  Product3/1 -> SumD2/2
  delta_P/1 -> Product2/1
  Product1/1 -> SumD2/1
  Ts/1 -> " "/1
  ref/1 -> Relational Operator/1
  val_unconstr/1 -> Relational Operator/2
  Relational Operator/1 -> " "/2

== system ECO_openSource/Controller/NMPC Algorithm/Subsystem/Algorithm/Calculate Initial Condition ==
  p : Inport
  Enable : EnablePort
  Calculate Condition at Start of Optimization : Subsystem
  Calculate Intake Condition : Subsystem
  Selector : Selector  InputPortWidth=6  IndexOptions=Index vector (dialog)  Indices=2  OutputSizes=1
  ux0 : Outport
  wires:
  Calculate Intake Condition/1(uxInt) -> Calculate Condition at Start of Optimization/1(uxInt)
  Calculate Condition at Start of Optimization/1(" ux0 ") -> ux0/1
  p/1 -> Selector/1, Calculate Condition at Start of Optimization/2(p)
  Selector/1 -> Calculate Intake Condition/1(pIM)

== system ECO_openSource/Controller/NMPC Algorithm/Subsystem/Algorithm/Create Bounds on h ==
  pMax : Inport
  dpMax : Inport  Port=2
  " Latest COC " : Constant  Value=-100
  " dpMax " : Constant  Value=-100
  " pMax " : Constant  Value=-100
  Extended repmat : MATLAB Function  TreatAsAtomicUnit=on
  Index of latest COC : Constant  Value=20
  Latest COC : Constant  Value=100
  Mux : Mux  Inputs=2
  Mux1 : Mux  Inputs=2
  Mux2 : Mux  Inputs=3
  Repmat : MATLAB Function  TreatAsAtomicUnit=on  mask{N=parECO.N}
  Scale Reference : Subsystem
  lh : Outport
  uh : Outport  Port=2
  wires:
  pMax/1 -> Mux/1
  dpMax/1 -> Mux/2
  Scale Reference/1(scaled) -> Mux1/1
  Mux/1 -> Scale Reference/1(unscaled)
  Latest COC/1 -> Mux1/2
  Mux1/1 -> Repmat/1(u)
  Mux2/1 -> Extended repmat/1(u)
  Index of latest COC/1 -> Extended repmat/2(idx)
  Extended repmat/1(y) -> lh/1
  Repmat/1(y) -> uh/1
  " Latest COC "/1 -> Mux2/3
  " dpMax "/1 -> Mux2/2
  " pMax "/1 -> Mux2/1

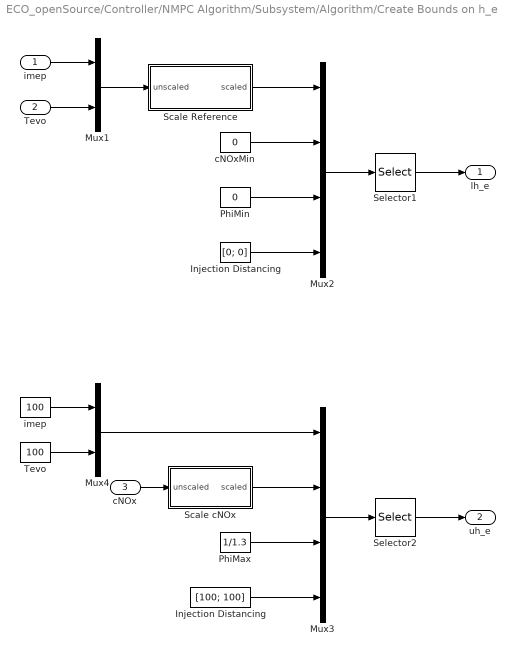
== system ECO_openSource/Controller/NMPC Algorithm/Subsystem/Algorithm/Create Bounds on h_e ==
  imep : Inport
  Tevo : Inport  Port=2
  cNOx : Inport  Port=3
  " Injection Distancing " : Constant  Value=[100; 100]
  " PhiMax " : Constant  Value=1/1.3
  " Tevo " : Constant  Value=100
  " imep " : Constant  Value=100
  Injection Distancing : Constant  Value=[0; 0]
  Mux1 : Mux  Inputs=2
  Mux2 : Mux
  Mux3 : Mux
  Mux4 : Mux  Inputs=2
  PhiMin : Constant  Value=0
  Scale Reference : Subsystem
  Scale cNOx : Subsystem
  Selector1 : Selector  InputPortWidth=6  IndexOptions=Index vector (dialog)  Indices=1:5  OutputSizes=1
  Selector2 : Selector  InputPortWidth=6  IndexOptions=Index vector (dialog)  Indices=1:5  OutputSizes=1
  cNOxMin : Constant  Value=0
  lh_e : Outport
  uh_e : Outport  Port=2
  wires:
  Scale Reference/1(scaled) -> Mux2/1
  Tevo/1 -> Mux1/2
  Mux1/1 -> Scale Reference/1(unscaled)
  imep/1 -> Mux1/1
  Mux2/1 -> Selector1/1
  Selector1/1 -> lh_e/1
  Mux4/1 -> Mux3/1
  " Tevo "/1 -> Mux4/2
  " imep "/1 -> Mux4/1
  Selector2/1 -> uh_e/1
  Mux3/1 -> Selector2/1
  PhiMin/1 -> Mux2/3
  Injection Distancing/1 -> Mux2/4
  cNOxMin/1 -> Mux2/2
  " Injection Distancing "/1 -> Mux3/4
  " PhiMax "/1 -> Mux3/3
  Scale cNOx/1(scaled) -> Mux3/2
  cNOx/1 -> Scale cNOx/1(unscaled)

== system ECO_openSource/Controller/NMPC Algorithm/Subsystem/Algorithm/Create Bounds on ux0 ==
  ux0Opt : Inport
  Mux3 : Mux  Inputs=2
  Mux4 : Mux  Inputs=2
  Selector : Selector  InputPortWidth=10  IndexOptions=Index vector (dialog)  Indices=5:10  OutputSizes=1
  lbu : Constant  Value=parECO.lbu
  ubu : Constant  Value=parECO.ubu
  lbux_0 : Outport
  ubux_0 : Outport  Port=2
  wires:
  Selector/1 -> Mux4/2, Mux3/2
  ubu/1 -> Mux4/1
  lbu/1 -> Mux3/1
  Mux3/1 -> lbux_0/1
  Mux4/1 -> ubux_0/1
  ux0Opt/1 -> Selector/1

== system ECO_openSource/Controller/NMPC Algorithm/Subsystem/Algorithm/Create ux_init ==
  ux0 : Inport
  p : Inport  Port=2
  Enable : EnablePort
  Subsystem : Subsystem
  Unscale ux0 : Subsystem
  ux_init : Outport
  wires:
  ux0/1 -> Unscale ux0/1(scaled)
  Subsystem/1(ux_init) -> ux_init/1
  Unscale ux0/1(unscaled) -> Subsystem/1(ux0)
  p/1 -> Subsystem/2(p)

== system ECO_openSource/Controller/NMPC Algorithm/Subsystem/Algorithm/Extract and Unscale Initial States and Inputs ==
  scaled : Inport
  Selector : Selector  IndexOptions=Index vector (dialog)  Indices=1:10  OutputSizes=1
  Sum : Sum  Inputs=|++
  offs : Constant  Value=[parECO.offsU; parECO.offsX; parECO.offsCA]
  scale : Gain  Gain=[parECO.scaleU; parECO.scaleX; parECO.scaleCA]
  unscaled : Outport
  wires:
  scale/1 -> Sum/1
  Sum/1 -> unscaled/1
  offs/1 -> Sum/2
  scaled/1 -> Selector/1
  Selector/1 -> scale/1

== system ECO_openSource/Controller/NMPC Algorithm/Subsystem/Algorithm/Model Simulation ==
  ux0 : Inport
  p : Inport  Port=2
  Constant : Constant  Value=parECO.dca_opt
  Constant1 : Constant  Value=parECO.dca_optAcados
  Create Outputs : Subsystem
  Delay1 : Delay  DelayLength=1  InitialConditionSource=Input port  InitialCondition=[parOpt.u0;parSim.OP.pInt;0;0]
      settings: InputPortMap=u0,p4
  For Iterator : ForIterator  ResetStates=reset  IterationLimit=parECO.N
  S-Function : S-Function  FunctionName=sfun_fsim  SFunctionDeploymentMode=off  EnableBusSupport=off
  Switch : Switch  Threshold=parECO.N-parECO.NAcados
  ySim : Outport
  wires:
  Constant/1 -> Switch/3
  Delay1/1 -> S-Function/1
  Constant1/1 -> Switch/1
  S-Function/2 -> Create Outputs/2(uxdot)  "uxdot"
  S-Function/1 -> Delay1/1, Create Outputs/1(ux)  "ux"
  Create Outputs/1(ySim) -> ySim/1
  For Iterator/1 -> Switch/2
  S-Function/3 -> Create Outputs/3(y)  "y"
  Switch/1 -> S-Function/3
  p/1 -> S-Function/2
  ux0/1 -> Delay1/2

== system ECO_openSource/Controller/NMPC Algorithm/Subsystem/Algorithm/Unscale ux0 ==
  scaled : Inport
  Sum : Sum  Inputs=|++
  offs : Constant  Value=[parECO.offsU;parECO.offsX;parECO.offsCA]
  scale : Gain  Gain=[parECO.scaleU;parECO.scaleX;parECO.scaleCA]
  unscaled : Outport
  wires:
  offs/1 -> Sum/2
  scaled/1 -> scale/1
  scale/1 -> Sum/1
  Sum/1 -> unscaled/1

== system ECO_openSource/Controller/NMPC Algorithm/Subsystem/Limit Reference and Reference Changes/Limit d_Tevo ==
  u[k] : Inport
  sim : Inport  Port=2
  u[k-1] : Inport  Port=3
  " " : Constant  Value=0  OutDataTypeStr=Inherit: Inherit via back propagation
  AND : Logic  AllPortsSameDT=off  OutDataTypeStr=boolean
  Add : Sum  Inputs=+-
  Add1 : Sum
  Compare To Constant : simulink/Logic and Bit Operations/Compare To Constant  relop=<=  const=274  OutDataTypeStr=boolean
  Delay : Delay  DelayLength=1  ExternalReset=Rising
      settings: InputPortMap=u0,r5
  NOT : Logic  Operator=NOT  AllPortsSameDT=off  OutDataTypeStr=boolean
  Saturation : Saturate  UpperLimit=10  LowerLimit=-100
  Sum : Sum  Inputs=|++
  Switch : Switch  Criteria=u2 > Threshold
  Switch1 : Switch  Criteria=u2 > Threshold
  Zero : Constant  OutDataTypeStr=Inherit: Inherit via back propagation
  y : Outport
  wires:
  u[k-1]/1 -> Add1/2, Add/2
  u[k]/1 -> Compare To Constant/1, Add/1
  Saturation/1 -> Add1/1
  Add/1 -> AND/2, Saturation/1
  Switch1/1 -> Sum/1
  Sum/1 -> Delay/1
  NOT/1 -> AND/1
  Zero/1 -> Switch1/1
  Switch/1 -> y/1
  AND/1 -> Switch1/2, Switch/2
  Delay/1 -> Sum/2, NOT/1
  " "/1 -> Switch1/3
  sim/1 -> Switch/1
  Add1/1 -> Switch/3
  Compare To Constant/1 -> Delay/2

== system ECO_openSource/Controller/NMPC Algorithm/Subsystem/Limit Reference and Reference Changes/Limit d_cNOx ==
  u[k] : Inport
  sim : Inport  Port=2
  u[k-1] : Inport  Port=3
  " " : Constant  Value=0  OutDataTypeStr=Inherit: Inherit via back propagation
  AND : Logic  AllPortsSameDT=off  OutDataTypeStr=boolean
  Add : Sum  Inputs=+-
  Add1 : Sum
  Compare To Constant : simulink/Logic and Bit Operations/Compare To Constant  relop=>=  const=9999  OutDataTypeStr=boolean
  Delay : Delay  DelayLength=1  ExternalReset=Rising
      settings: InputPortMap=u0,r5
  NOT : Logic  Operator=NOT  AllPortsSameDT=off  OutDataTypeStr=boolean
  Saturation : Saturate  UpperLimit=50  LowerLimit=-50
  Sum : Sum  Inputs=|++
  Switch : Switch  Criteria=u2 > Threshold
  Switch1 : Switch  Criteria=u2 > Threshold
  Zero : Constant  OutDataTypeStr=Inherit: Inherit via back propagation
  y : Outport
  wires:
  u[k-1]/1 -> Add1/2, Add/2
  u[k]/1 -> Compare To Constant/1, Add/1
  Saturation/1 -> Add1/1
  Add/1 -> AND/2, Saturation/1
  Switch1/1 -> Sum/1
  Sum/1 -> Delay/1
  NOT/1 -> AND/1
  Zero/1 -> Switch1/1
  Switch/1 -> y/1
  AND/1 -> Switch1/2, Switch/2
  Delay/1 -> Sum/2, NOT/1
  " "/1 -> Switch1/3
  sim/1 -> Switch/1
  Add1/1 -> Switch/3
  Compare To Constant/1 -> Delay/2

== system ECO_openSource/Controller/NMPC Algorithm/Subsystem/Limit Reference and Reference Changes/Limit d_dpMax ==
  u[k] : Inport
  sim : Inport  Port=2
  u[k-1] : Inport  Port=3
  " " : Constant  Value=0  OutDataTypeStr=Inherit: Inherit via back propagation
  AND : Logic  AllPortsSameDT=off  OutDataTypeStr=boolean
  Add : Sum  Inputs=+-
  Add1 : Sum
  Compare To Constant : simulink/Logic and Bit Operations/Compare To Constant  relop=>=  const=14e5  OutDataTypeStr=boolean
  Delay : Delay  DelayLength=1  ExternalReset=Rising
      settings: InputPortMap=u0,r5
  NOT : Logic  Operator=NOT  AllPortsSameDT=off  OutDataTypeStr=boolean
  Saturation : Saturate  UpperLimit=0.5e5  LowerLimit=-0.5e5
  Sum : Sum  Inputs=|++
  Switch : Switch  Criteria=u2 > Threshold
  Switch1 : Switch  Criteria=u2 > Threshold
  Zero : Constant  OutDataTypeStr=Inherit: Inherit via back propagation
  y : Outport
  wires:
  Switch/1 -> y/1
  NOT/1 -> AND/1
  Switch1/1 -> Sum/1
  Delay/1 -> NOT/1, Sum/2
  Add1/1 -> Switch/3
  Add/1 -> AND/2, Saturation/1
  u[k-1]/1 -> Add1/2, Add/2
  Sum/1 -> Delay/1
  Zero/1 -> Switch1/1
  AND/1 -> Switch1/2, Switch/2
  sim/1 -> Switch/1
  " "/1 -> Switch1/3
  u[k]/1 -> Compare To Constant/1, Add/1
  Saturation/1 -> Add1/1
  Compare To Constant/1 -> Delay/2

== system ECO_openSource/Controller/NMPC Algorithm/Subsystem/Limit Reference and Reference Changes/Limit d_imep ==
  u[k] : Inport
  u[k-1] : Inport  Port=2
  Add : Sum  Inputs=+-
  Add1 : Sum
  Saturation : Saturate  UpperLimit=0.5e5  LowerLimit=-0.5e5
  y : Outport
  wires:
  u[k-1]/1 -> Add1/2, Add/2
  u[k]/1 -> Add/1
  Add/1 -> Saturation/1
  Saturation/1 -> Add1/1
  Add1/1 -> y/1

== system ECO_openSource/Controller/NMPC Algorithm/Subsystem/Algorithm/Calculate Initial Condition/Calculate Condition at Start of Optimization ==
  uxInt : Inport
  p : Inport  Port=2
  Delay1 : Delay  DelayLength=1  InitialConditionSource=Input port  InitialCondition=[parOpt.u0;parSim.OP.pInt;0;0]
      settings: InputPortMap=u0,p4
  For Iterator : ForIterator  ResetStates=reset  IterationLimit=numel(parECO.ca_x0Opt)-1  ShowIterationPort=off
  S-Function : S-Function  FunctionName=sfun_fsim  SFunctionDeploymentMode=off  EnableBusSupport=off
  Scale ux0 : Subsystem
  Terminator : Terminator
  Terminator2 : Terminator
  dca : Constant  Value=parECO.dca_x0Opt
  " ux0 " : Outport
  wires:
  Delay1/1 -> S-Function/1
  S-Function/1 -> Delay1/1, Scale ux0/1(unscaled)  "ux"
  uxInt/1 -> Delay1/2
  Scale ux0/1(scaled) -> " ux0 "/1
  S-Function/2 -> Terminator/1  "uxdot"
  S-Function/3 -> Terminator2/1  "y"
  dca/1 -> S-Function/3
  p/1 -> S-Function/2

== system ECO_openSource/Controller/NMPC Algorithm/Subsystem/Algorithm/Calculate Initial Condition/Calculate Intake Condition ==
  pIM : Inport
  Constant : Constant  Value=-7122.9
  Constant1 : Constant  Value=parECO.u0
  Constant2 : Constant  Value=parECO.ca_ivc
  Constant3 : Constant  Value=0
  Constant4 : Constant  Value=0
  Constant5 : Constant  Value=382
  Constant6 : Constant  Value=0
  Gain : Gain  Gain=1.1517
  Mux : Mux  Inputs=3
  Mux1 : Mux  Inputs=5
  Sum : Sum  Inputs=|++
  uxInt : Outport
  wires:
  Gain/1 -> Sum/1
  Constant/1 -> Sum/2
  pIM/1 -> Gain/1
  Mux1/1 -> Mux/2  "x0"
  Constant1/1 -> Mux/1  "u0"
  Sum/1 -> Mux1/1  "pInt"
  Constant3/1 -> Mux1/2  "QcInt"
  Constant4/1 -> Mux1/3  "wInt"
  Mux/1 -> uxInt/1
  Constant2/1 -> Mux/3  "ca_ivc"
  Constant5/1 -> Mux1/4  "thetaInt"
  Constant6/1 -> Mux1/5  "cNOxInt"

== system ECO_openSource/Controller/NMPC Algorithm/Subsystem/Algorithm/Create Bounds on h/Scale Reference ==
  unscaled : Inport
  Sum : Sum  Inputs=|+-
  offs : Constant  Value=[parECO.offsX(1); 0]
  scale : Gain  Gain=1./(ones(2,1)*parECO.scaleX(1))
  scaled : Outport
  wires:
  offs/1 -> Sum/2
  unscaled/1 -> Sum/1
  Sum/1 -> scale/1
  scale/1 -> scaled/1
